simulink model "shortPeriodSimulink"  (R2016b)
settings: Solver=FixedStepAuto  StartTime=0.0  StopTime=10  FixedStep=0.0025  RelTol=1e-3
values from neighbouring files (symbols this model uses):
  A = [ ... (first row only)    [allPeriod.m]    (also in shortPeriod.m)
  B = [ ... (first row only)    [allPeriod.m]    (also in shortPeriod.m)
  C_L_alpha = 4.44    [allPeriod.m]    (also in shortPeriod.m)
  g = 9.81    [allPeriod.m]    (also in shortPeriod.m)
  q_star = rho * (V_star)^2/2    (= 1767.57602)    [allPeriod.m]    (also in shortPeriod.m)
  S = 17.1    [allPeriod.m]    (also in shortPeriod.m)
  V_co = 122    [allPeriod.m]    (also in shortPeriod.m)
  W = 12224    [allPeriod.m]    (also in shortPeriod.m)
settings Model: Creator=admin  LastModifiedBy=admin

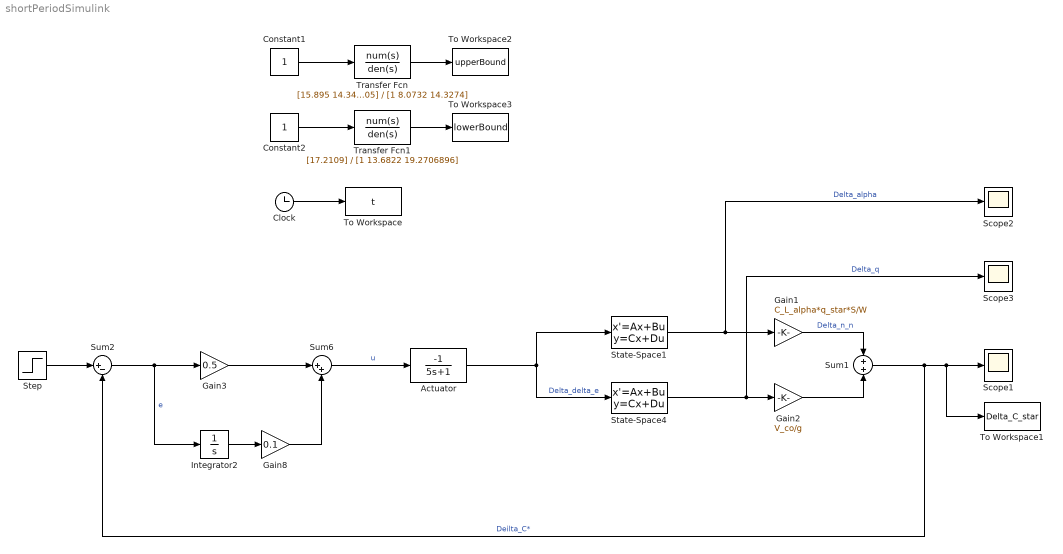
== system shortPeriodSimulink ==
  "Actuator " : TransferFcn  Numerator=[-1]  Denominator=[5 1]
  Clock : Clock
  Constant1 : Constant
  Constant2 : Constant
  Gain1 : Gain  Gain=C_L_alpha*q_star*S/W
      mask Display: disp('K_\alpha','texmode','on');
  Gain2 : Gain  Gain=V_co/g
      mask Display: disp('K_q','texmode','on');
  Gain3 : Gain  Gain=0.5
      mask Display: disp('K_P','texmode','on');
  Gain8 : Gain  Gain=0.1
      mask Display: disp('K_I','texmode','on');
  Integrator2 : Integrator
  Scope1 : Scope
  Scope2 : Scope
  Scope3 : Scope
  State-Space1 : StateSpace  A=A  B=B  C=[1 0]  D=0  X0=0
  State-Space4 : StateSpace  A=A  B=B  C=[0 1]  D=0  X0=0
  Step : Step  Time=0  SampleTime=0
  Sum1 : Sum  Inputs=+|+
  Sum2 : Sum  Inputs=|+-
  Sum6 : Sum  Inputs=|++
  To Workspace : ToWorkspace  VariableName=t  SampleTime=-1
  To Workspace1 : ToWorkspace  VariableName=Delta_C_star  SampleTime=-1
      mask Display: disp('\DeltaC*','texmode','on');
  To Workspace2 : ToWorkspace  VariableName=upperBound  SampleTime=-1
  To Workspace3 : ToWorkspace  VariableName=lowerBound  SampleTime=-1
  Transfer Fcn : TransferFcn  Numerator=[15.895 14.3405]  Denominator=[1 8.0732 14.3274]
  Transfer Fcn1 : TransferFcn  Numerator=[17.2109]  Denominator=[1 13.6822 19.2706896]
  wires:
  State-Space1/1 -> Gain1/1, Scope2/1  "Delta_alpha"
  State-Space4/1 -> Gain2/1, Scope3/1  "Delta_q"
  Sum2/1 -> Integrator2/1, Gain3/1  "e"
  Sum6/1 -> "Actuator "/1  "u"
  Integrator2/1 -> Gain8/1
  Gain8/1 -> Sum6/2
  Gain3/1 -> Sum6/1
  "Actuator "/1 -> State-Space4/1, State-Space1/1  "Delta_delta_e"
  Step/1 -> Sum2/1
  Gain1/1 -> Sum1/1  "Delta_n_n"
  Gain2/1 -> Sum1/2
  Sum1/1 -> To Workspace1/1, Scope1/1, Sum2/2  "Deilta_C*"
  Clock/1 -> To Workspace/1
  Constant1/1 -> Transfer Fcn/1
  Constant2/1 -> Transfer Fcn1/1
  Transfer Fcn/1 -> To Workspace2/1
  Transfer Fcn1/1 -> To Workspace3/1
